simulink model "GFLIB_Ramp_BAM_FLT"  (Simulink 8.3)
settings: Solver=ode45  StartTime=0.0  StopTime=10.0  RelTol=1e-3
undefined symbols (not defined in the file): fltRampDown, fltRampUp
settings Model: Creator=B17364  LastModifiedBy=B17364
settings OptimizationCC: ExpressionDepthLimit=2147483647
settings DebuggingCC: FcnCallInpInsideContextMsg=UseLocalSettings  StrictBusMsg=Warning

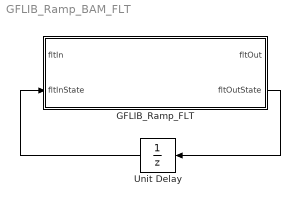
== system GFLIB_Ramp_BAM_FLT ==
  GFLIB_Ramp_FLT : Subsystem  mask(GFLIB_Ramp){fltRampUp=fltRampUp, fltRampDown=fltRampDown}
      mask help: Bit accurate model of ramp function. All parameters as well as input and output are in single precision floating data format.
      mask init:
      | pos = get_param(gcb, 'Position');width = pos(3) - pos(1); height = pos(4) - pos(2);tX=width/2;tY=height*0.9;
      mask Display: color('black');port_label('input',1,'fltIn');port_label('input',2,'fltInState');port_label('output',1,'fltOut');port_label('output',2,'fltOutState');color('black');disp('GFLIB_Ramp_FLT');color('blue');text(tX,tY, 'BAM', 'horizontalAlignment', 'center');
  Unit Delay : UnitDelay  SampleTime=-1
  wires:
  GFLIB_Ramp_FLT/2(fltOutState) -> Unit Delay/1
  Unit Delay/1 -> GFLIB_Ramp_FLT/2(fltInState)

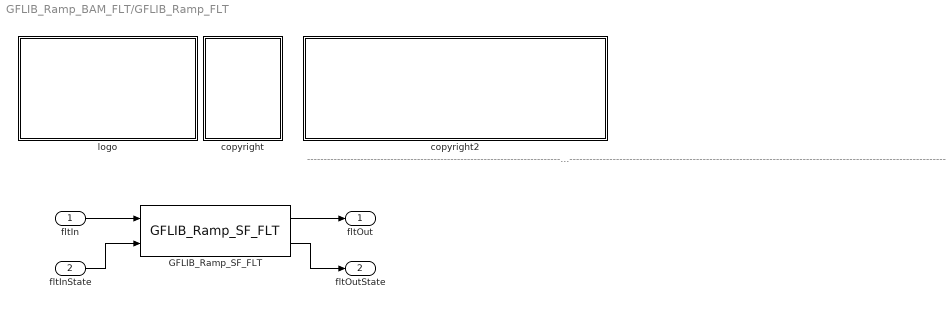
== system GFLIB_Ramp_BAM_FLT/GFLIB_Ramp_FLT ==
  note: ---------------------------------------------------------------------------------------------------------------------------------------------------------------------------------------------------
  fltIn : Inport
  fltInState : Inport  Port=2
  GFLIB_Ramp_SF_FLT : S-Function  FunctionName=GFLIB_Ramp_SF_FLT  Parameters=fltRampUp,fltRampDown  EnableBusSupport=off
  copyright : Subsystem
      mask Display:
      | text(10,90,'FILE:');text(10,75,'DESRIPTION:')
      | text(10,60,'COPYRIGHT:')
      | text(10,45,'VERSION:')
      | text(10,30,'DATE:')
      | text(10,15,'AUTHOR:')
  copyright2 : Subsystem
      mask Display:
      | text(10,90,'GFLIB_Ramp_BAM_FLT.mdl');text(10,75,'Rate of change limiter - Ramp function.');text(10,60,'Freescale')
      | text(10,45,'0.1');text(10,30,'08-Apr-2014');text(10,15,'');
  logo : Subsystem
      mask Display: image(imread('logo.jpg'))
  fltOut : Outport
  fltOutState : Outport  Port=2
  wires:
  fltIn/1 -> GFLIB_Ramp_SF_FLT/1
  GFLIB_Ramp_SF_FLT/1 -> fltOut/1
  fltInState/1 -> GFLIB_Ramp_SF_FLT/2
  GFLIB_Ramp_SF_FLT/2 -> fltOutState/1

== system GFLIB_Ramp_BAM_FLT/GFLIB_Ramp_FLT/copyright ==

== system GFLIB_Ramp_BAM_FLT/GFLIB_Ramp_FLT/copyright2 ==

== system GFLIB_Ramp_BAM_FLT/GFLIB_Ramp_FLT/logo ==
